simulink model "example1"  (R2015a)
settings: Solver=ode45  StartTime=0.0  StopTime=inf  RelTol=1e-3
settings Model: Creator=Teme  LastModifiedBy=teme

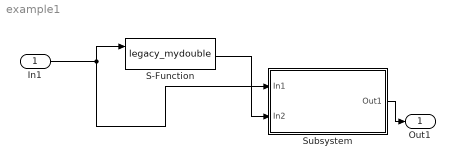
== system example1 ==
  In1 : Inport
  S-Function : S-Function  FunctionName=legacy_mydouble
  Subsystem : Subsystem
  Out1 : Outport
  wires:
  S-Function/1 -> Subsystem/2(In2)
  Subsystem/1(Out1) -> Out1/1
  In1/1 -> Subsystem/1(In1), S-Function/1

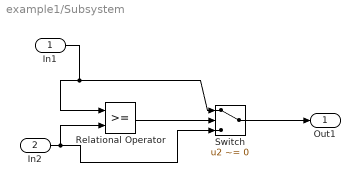
== system example1/Subsystem ==
  In1 : Inport
  In2 : Inport  Port=2
  Relational Operator : RelationalOperator  OutDataTypeStr=boolean
  Switch : Switch  Criteria=u2 ~= 0
  Out1 : Outport
  wires:
  In1/1 -> Relational Operator/1, Switch/1
  In2/1 -> Relational Operator/2, Switch/3
  Relational Operator/1 -> Switch/2
  Switch/1 -> Out1/1
